simulink model "two"  (R2020b)
settings: Solver=VariableStepAuto  StartTime=0.0  StopTime=100  RelTol=1e-3
values from neighbouring files (symbols this model uses):
  b = 10    [variable.m]
  k1 = 20    [variable.m]
  k2 = 30    [variable.m]
  m1 = 500    [variable.m]
  m2 = 50    [variable.m]
settings Model: Creator=USER  LastModifiedBy=USER

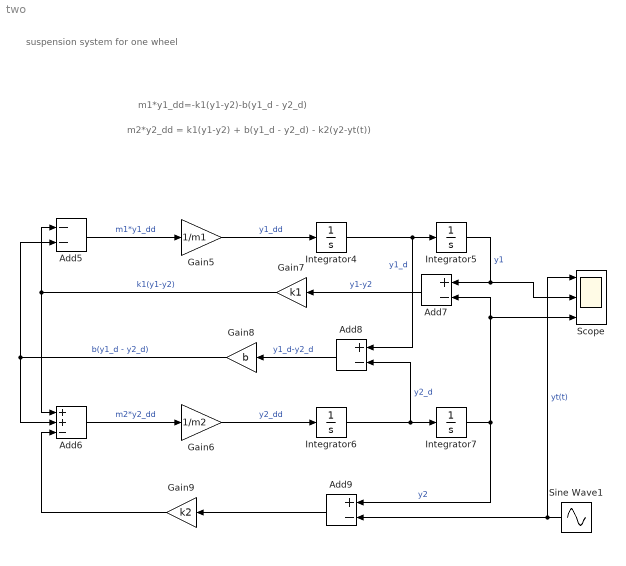
== system two ==
  note: m2*y2_dd = k1(y1-y2) + b(y1_d - y2_d) - k2(y2-yt(t))
  note: m1*y1_dd=-k1(y1-y2)-b(y1_d - y2_d)
  note: suspension system for one wheel
  Add5 : Sum  Inputs=--
  Add6 : Sum  Inputs=++-
  Add7 : Sum  Inputs=+-
  Add8 : Sum  Inputs=+-
  Add9 : Sum  Inputs=+-
  Gain5 : Gain  Gain=1/m1
  Gain6 : Gain  Gain=1/m2
  Gain7 : Gain  Gain=k1
  Gain8 : Gain  Gain=b
  Gain9 : Gain  Gain=k2
  Integrator{4..7} (4 alike) : Integrator
  Scope : Scope  NumInputPorts=3
  Sine Wave1 : Sin  SampleTime=0
  wires:
  Add5/1 -> Gain5/1  "m1*y1_dd"
  Gain5/1 -> Integrator4/1  "y1_dd"
  Integrator4/1 -> Add8/1, Integrator5/1  "y1_d"
  Integrator5/1 -> Scope/2, Add7/1  "y1"
  Add6/1 -> Gain6/1  "m2*y2_dd"
  Gain6/1 -> Integrator6/1  "y2_dd"
  Integrator6/1 -> Add8/2, Integrator7/1  "y2_d"
  Integrator7/1 -> Add9/1, Add7/2, Scope/3  "y2"
  Add7/1 -> Gain7/1  "y1-y2"
  Gain7/1 -> Add6/1, Add5/1  "k1(y1-y2)"
  Add8/1 -> Gain8/1  "y1_d-y2_d"
  Gain8/1 -> Add6/2, Add5/2  "b(y1_d - y2_d)"
  Gain9/1 -> Add6/3
  Add9/1 -> Gain9/1
  Sine Wave1/1 -> Scope/1, Add9/2  "yt(t)"
